simulink model "sumilink"  (R2016a)
settings: Solver=VariableStepAuto  StartTime=0.0  StopTime=2  RelTol=1e-3
values from neighbouring files (symbols this model uses):
  B = fm+(km^2/R)    (= 0.0793582758621)    [saadimfile.m]
  b1 = 0.25    [saadimfile.m]
  b2 = 0.25    [saadimfile.m]
  g = 10    [saadimfile.m]
  K = km/(N*R)    (= 0.00164482758621)    [saadimfile.m]
  k = 0.5    [saadimfile.m]
  l = 0.2    [saadimfile.m]
  M11 = M(1,1)    [saadimfile.m]
  M12 = M(1,2)    [saadimfile.m]
  m2 = 1    [saadimfile.m]
  M22 = M(2,2)    [saadimfile.m]
  N = 50    [saadimfile.m]
libraries: simulink x4
settings Model: Creator=USER  LastModifiedBy=USER

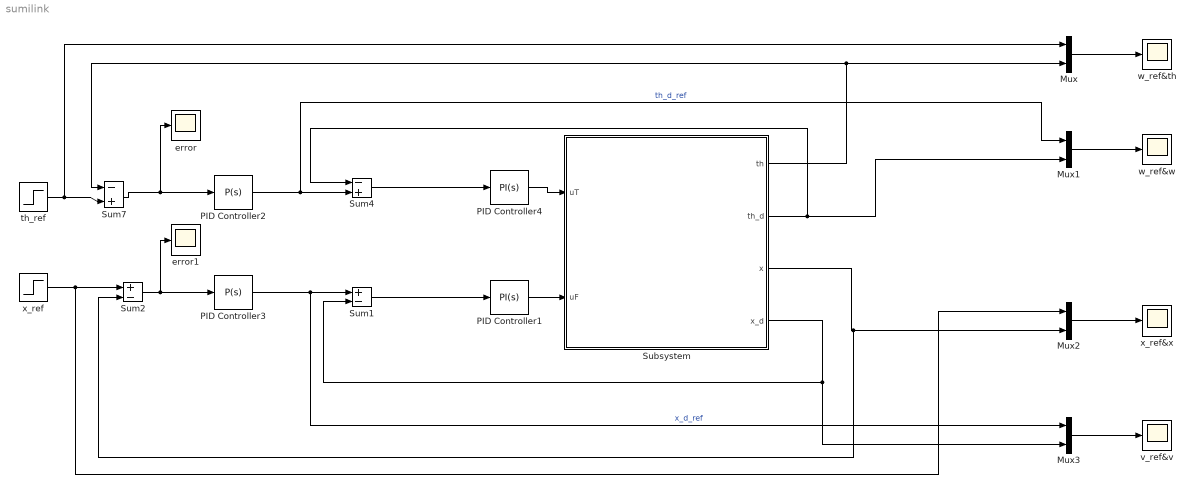
== system sumilink ==
  Mux{,1..3} (4 alike) : Mux  Inputs=2
  PID Controller1 : simulink/Continuous/PID Controller  Controller=PI  TimeDomain=Continuous-time  SampleTime=-1  IntegratorMethod=Forward Euler  FilterMethod=Forward Euler  Form=Parallel  UseFilter=on  ControllerParametersSource=internal  P=4000  I=150  D=0  N=100  InitialConditionSource=internal  InitialConditionForIntegrator=0  InitialConditionForFilter=0  ExternalReset=none  LimitOutput=off  UpperSaturationLimit=inf  LowerSaturationLimit=-inf  LinearizeAsGain=on  AntiWindupMode=none  Kb=1  TrackingMode=off  Kt=1  PParamMin=[]  PParamMax=[]  IParamMin=[]  IParamMax=[]  DParamMin=[]  DParamMax=[]  NParamMin=[]  NParamMax=[]  KbParamMin=[]  KbParamMax=[]  KtParamMin=[]  KtParamMax=[]  POutMin=[]  POutMax=[]  IOutMin=[]  IOutMax=[]  DOutMin=[]  DOutMax=[]  NOutMin=[]  NOutMax=[]  KbOutMin=[]  KbOutMax=[]  KtOutMin=[]  KtOutMax=[]  IntegratorOutMin=[]  IntegratorOutMax=[]  FilterOutMin=[]  FilterOutMax=[]  SumOutMin=[]  SumOutMax=[]  SumI1OutMin=[]  SumI1OutMax=[]  SumI2OutMin=[]  SumI2OutMax=[]  SumI3OutMin=[]  SumI3OutMax=[]  SumDOutMin=[]  SumDOutMax=[]  SaturationOutMin=[]  SaturationOutMax=[]  IntegratorContinuousStateAttributes=''  IntegratorStateMustResolveToSignalObject=off  IntegratorRTWStateStorageClass=Auto  FilterContinuousStateAttributes=''  FilterStateMustResolveToSignalObject=off  FilterRTWStateStorageClass=Auto  DifferentiatorICPrevScaledInput=0  DifferentiatorOutMin=[]  DifferentiatorOutMax=[]
  PID Controller2 : simulink/Continuous/PID Controller  Controller=P  TimeDomain=Continuous-time  SampleTime=-1  IntegratorMethod=Forward Euler  FilterMethod=Forward Euler  Form=Parallel  UseFilter=on  ControllerParametersSource=internal  P=120  I=1  D=0  N=100  InitialConditionSource=internal  InitialConditionForIntegrator=0  InitialConditionForFilter=0  ExternalReset=none  LimitOutput=off  UpperSaturationLimit=inf  LowerSaturationLimit=-inf  LinearizeAsGain=on  AntiWindupMode=none  Kb=1  TrackingMode=off  Kt=1  PParamMin=[]  PParamMax=[]  IParamMin=[]  IParamMax=[]  DParamMin=[]  DParamMax=[]  NParamMin=[]  NParamMax=[]  KbParamMin=[]  KbParamMax=[]  KtParamMin=[]  KtParamMax=[]  POutMin=[]  POutMax=[]  IOutMin=[]  IOutMax=[]  DOutMin=[]  DOutMax=[]  NOutMin=[]  NOutMax=[]  KbOutMin=[]  KbOutMax=[]  KtOutMin=[]  KtOutMax=[]  IntegratorOutMin=[]  IntegratorOutMax=[]  FilterOutMin=[]  FilterOutMax=[]  SumOutMin=[]  SumOutMax=[]  SumI1OutMin=[]  SumI1OutMax=[]  SumI2OutMin=[]  SumI2OutMax=[]  SumI3OutMin=[]  SumI3OutMax=[]  SumDOutMin=[]  SumDOutMax=[]  SaturationOutMin=[]  SaturationOutMax=[]  IntegratorContinuousStateAttributes=''  IntegratorStateMustResolveToSignalObject=off  IntegratorRTWStateStorageClass=Auto  FilterContinuousStateAttributes=''  FilterStateMustResolveToSignalObject=off  FilterRTWStateStorageClass=Auto  DifferentiatorICPrevScaledInput=0  DifferentiatorOutMin=[]  DifferentiatorOutMax=[]
  PID Controller3 : simulink/Continuous/PID Controller  Controller=P  TimeDomain=Continuous-time  SampleTime=-1  IntegratorMethod=Forward Euler  FilterMethod=Forward Euler  Form=Parallel  UseFilter=on  ControllerParametersSource=internal  P=75  I=1  D=0  N=100  InitialConditionSource=internal  InitialConditionForIntegrator=0  InitialConditionForFilter=0  ExternalReset=none  LimitOutput=off  UpperSaturationLimit=inf  LowerSaturationLimit=-inf  LinearizeAsGain=on  AntiWindupMode=none  Kb=1  TrackingMode=off  Kt=1  PParamMin=[]  PParamMax=[]  IParamMin=[]  IParamMax=[]  DParamMin=[]  DParamMax=[]  NParamMin=[]  NParamMax=[]  KbParamMin=[]  KbParamMax=[]  KtParamMin=[]  KtParamMax=[]  POutMin=[]  POutMax=[]  IOutMin=[]  IOutMax=[]  DOutMin=[]  DOutMax=[]  NOutMin=[]  NOutMax=[]  KbOutMin=[]  KbOutMax=[]  KtOutMin=[]  KtOutMax=[]  IntegratorOutMin=[]  IntegratorOutMax=[]  FilterOutMin=[]  FilterOutMax=[]  SumOutMin=[]  SumOutMax=[]  SumI1OutMin=[]  SumI1OutMax=[]  SumI2OutMin=[]  SumI2OutMax=[]  SumI3OutMin=[]  SumI3OutMax=[]  SumDOutMin=[]  SumDOutMax=[]  SaturationOutMin=[]  SaturationOutMax=[]  IntegratorContinuousStateAttributes=''  IntegratorStateMustResolveToSignalObject=off  IntegratorRTWStateStorageClass=Auto  FilterContinuousStateAttributes=''  FilterStateMustResolveToSignalObject=off  FilterRTWStateStorageClass=Auto  DifferentiatorICPrevScaledInput=0  DifferentiatorOutMin=[]  DifferentiatorOutMax=[]
  PID Controller4 : simulink/Continuous/PID Controller  Controller=PI  TimeDomain=Continuous-time  SampleTime=-1  IntegratorMethod=Forward Euler  FilterMethod=Forward Euler  Form=Parallel  UseFilter=on  ControllerParametersSource=internal  P=6000  I=150  D=0  N=100  InitialConditionSource=internal  InitialConditionForIntegrator=0  InitialConditionForFilter=0  ExternalReset=none  LimitOutput=off  UpperSaturationLimit=inf  LowerSaturationLimit=-inf  LinearizeAsGain=on  AntiWindupMode=none  Kb=1  TrackingMode=off  Kt=1  PParamMin=[]  PParamMax=[]  IParamMin=[]  IParamMax=[]  DParamMin=[]  DParamMax=[]  NParamMin=[]  NParamMax=[]  KbParamMin=[]  KbParamMax=[]  KtParamMin=[]  KtParamMax=[]  POutMin=[]  POutMax=[]  IOutMin=[]  IOutMax=[]  DOutMin=[]  DOutMax=[]  NOutMin=[]  NOutMax=[]  KbOutMin=[]  KbOutMax=[]  KtOutMin=[]  KtOutMax=[]  IntegratorOutMin=[]  IntegratorOutMax=[]  FilterOutMin=[]  FilterOutMax=[]  SumOutMin=[]  SumOutMax=[]  SumI1OutMin=[]  SumI1OutMax=[]  SumI2OutMin=[]  SumI2OutMax=[]  SumI3OutMin=[]  SumI3OutMax=[]  SumDOutMin=[]  SumDOutMax=[]  SaturationOutMin=[]  SaturationOutMax=[]  IntegratorContinuousStateAttributes=''  IntegratorStateMustResolveToSignalObject=off  IntegratorRTWStateStorageClass=Auto  FilterContinuousStateAttributes=''  FilterStateMustResolveToSignalObject=off  FilterRTWStateStorageClass=Auto  DifferentiatorICPrevScaledInput=0  DifferentiatorOutMin=[]  DifferentiatorOutMax=[]
  Subsystem : Subsystem
  Sum1 : Sum  Inputs=+-
  Sum2 : Sum  Inputs=+-
  Sum4 : Sum  Inputs=-+
  Sum7 : Sum  Inputs=-+
  error : Scope
  error1 : Scope
  th_ref : Step  After=pi/3  SampleTime=0
  v_ref&v : Scope
  w_ref&th : Scope
  w_ref&w : Scope
  x_ref : Step  After=10  SampleTime=0
  x_ref&x : Scope
  wires:
  PID Controller4/1 -> Subsystem/1(uT)
  PID Controller3/1 -> Mux3/1, Sum1/1  "x_d_ref"
  th_ref/1 -> Mux/1, Sum7/2
  Sum1/1 -> PID Controller1/1
  PID Controller1/1 -> Subsystem/2(uF)
  Sum2/1 -> error1/1, PID Controller3/1
  Sum7/1 -> PID Controller2/1, error/1
  Mux/1 -> w_ref&th/1
  Mux1/1 -> w_ref&w/1
  Mux2/1 -> x_ref&x/1
  Mux3/1 -> v_ref&v/1
  Subsystem/1(th) -> Sum7/1, Mux/2
  Subsystem/2(th_d) -> Sum4/1, Mux1/2
  Subsystem/3(x) -> Sum2/2, Mux2/2
  x_ref/1 -> Mux2/1, Sum2/1
  Subsystem/4(x_d) -> Sum1/2, Mux3/2
  PID Controller2/1 -> Mux1/1, Sum4/2  "th_d_ref"
  Sum4/1 -> PID Controller4/1

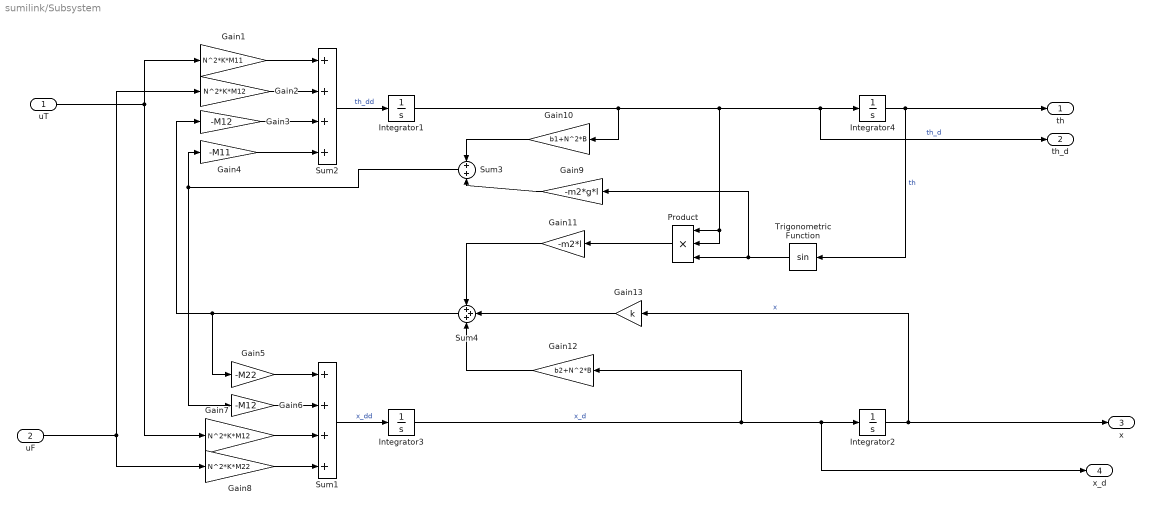
== system sumilink/Subsystem ==
  uT : Inport
  uF : Inport  Port=2
  Gain1 : Gain  Gain=N^2*K*M11
  Gain10 : Gain  Gain=b1+N^2*B
  Gain11 : Gain  Gain=-m2*l
  Gain12 : Gain  Gain=b2+N^2*B
  Gain13 : Gain  Gain=k
  Gain2 : Gain  Gain=N^2*K*M12
  Gain3 : Gain  Gain=-M12
  Gain4 : Gain  Gain=-M11
  Gain5 : Gain  Gain=-M22
  Gain6 : Gain  Gain=-M12
  Gain7 : Gain  Gain=N^2*K*M12
  Gain8 : Gain  Gain=N^2*K*M22
  Gain9 : Gain  Gain=-m2*g*l
  Integrator{1..4} (4 alike) : Integrator
  Product : Product  Inputs=3
  Sum1 : Sum  Inputs=4
  Sum2 : Sum  Inputs=4
  Sum3 : Sum  Inputs=2
  Sum4 : Sum  Inputs=3
  Trigonometric Function : Trigonometry
  th : Outport
  th_d : Outport  Port=2
  x : Outport  Port=3
  x_d : Outport  Port=4
  wires:
  Integrator4/1 -> th/1, Trigonometric Function/1  "th"
  Integrator2/1 -> x/1, Gain13/1  "x"
  Integrator3/1 -> Gain12/1, x_d/1, Integrator2/1  "x_d"
  Integrator1/1 -> Gain10/1, Product/1, Product/2, th_d/1, Integrator4/1  "th_d"
  Gain12/1 -> Sum4/3
  uT/1 -> Gain7/1, Gain1/1
  Product/1 -> Gain11/1
  Gain10/1 -> Sum3/1
  Gain9/1 -> Sum3/2
  uF/1 -> Gain2/1, Gain8/1
  Gain4/1 -> Sum2/4
  Gain3/1 -> Sum2/3
  Trigonometric Function/1 -> Gain9/1, Product/3
  Gain7/1 -> Sum1/3
  Sum3/1 -> Gain4/1, Gain6/1
  Sum4/1 -> Gain5/1, Gain3/1
  Gain11/1 -> Sum4/1
  Gain6/1 -> Sum1/2
  Gain5/1 -> Sum1/1
  Gain13/1 -> Sum4/2
  Gain8/1 -> Sum1/4
  Gain1/1 -> Sum2/1
  Sum2/1 -> Integrator1/1  "th_dd"
  Sum1/1 -> Integrator3/1  "x_dd"
  Gain2/1 -> Sum2/2
